simulink model "Timestamp_delta_Sysobj_model"  (R2021b)
settings: Solver=FixedStepAuto  StartTime=0.0  StopTime=50  RelTol=1e-3
settings Model: Creator=kilyovsk  LastModifiedBy=kilyovsk
settings SolverCC: ConcurrentTasks=on  PositivePriorityOrder=on
settings OptimizationCC: BlockReduction=off  OptimizeBlockIOStorage=off
settings DebuggingCC: TasksWithSamePriorityMsg=none
settings HardwareCC: ProdBitPerLong=64  ProdLongLongMode=on  ProdHWDeviceType=Intel->x86-64 (Linux 64)
settings SFSimCC: SimCustomHeaderCode=|
  | #include "findDelta.h"
  | #include "getTime.h"
settings SFSimCC: SimUserSources=|
  | findDelta_script.c
  | getTime_script.c
settings RTWCC: Description=Simulink Real-Time  SystemTargetFile=slrealtime.tlc  TemplateMakefile=slrealtime_default_tmf  Toolchain=Simulink Real-Time Toolchain  BuildConfiguration=Faster Runs  CodeExecutionProfiling=on  TargetLang=C++
settings RTWCC: CustomHeaderCode=|
  | #include "findDelta.h"
  | #include "getTime.h"
settings RTWCC: CustomSource=|
  | findDelta_script.c
  | getTime_script.c

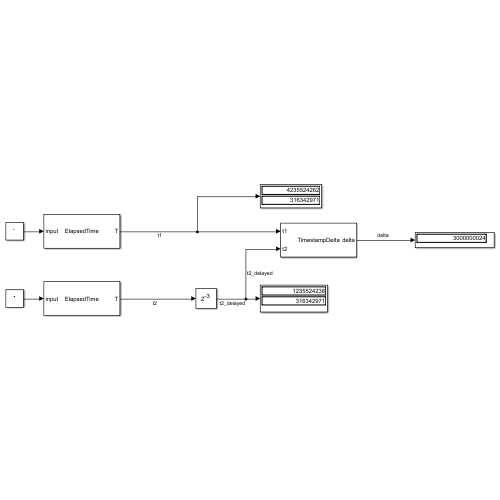
[thumbnail: Simulink's stored preview of the top-level diagram]
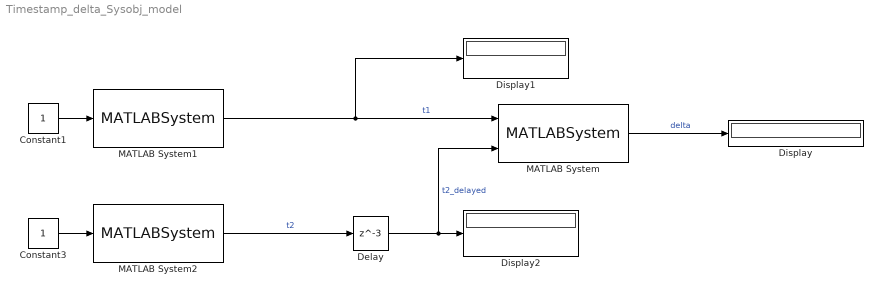
== system Timestamp_delta_Sysobj_model ==
  Constant1 : Constant
  Constant3 : Constant
  Delay : Delay  DelayLength=3  InitialCondition=0
  Display : Display
  Display1 : Display
  Display2 : Display
  MATLAB System : MATLABSystem  System=TimestampDelta  SimulateUsing=Code generation
      mask Type: TimestampDelta
      mask Display:
      | disp('TimestampDelta');
      | port_label('input',1,'t1');
      | port_label('input',2,'t2');
      | port_label('output',1,'delta');
  MATLAB System1 : MATLABSystem  System=ElapsedTime  SimulateUsing=Code generation
      mask Type: ElapsedTime
      mask Display:
      | disp('ElapsedTime');
      | port_label('input',1,'input');
      | port_label('output',1,'T');
  MATLAB System2 : MATLABSystem  System=ElapsedTime  SimulateUsing=Code generation
      mask Type: ElapsedTime
      mask Display:
      | disp('ElapsedTime');
      | port_label('input',1,'input');
      | port_label('output',1,'T');
  wires:
  MATLAB System1/1 -> Display1/1, MATLAB System/1  "t1"
  Delay/1 -> MATLAB System/2, Display2/1  "t2_delayed"
  Constant1/1 -> MATLAB System1/1
  Constant3/1 -> MATLAB System2/1
  MATLAB System/1 -> Display/1  "delta"
  MATLAB System2/1 -> Delay/1  "t2"
